simulink library "halout"  (R2021b)
settings: Solver=VariableStepAuto  StartTime=0.0  StopTime=10.0  RelTol=1e-3
undefined symbols (not defined in the file): C_TASK_5MS_S, FALSE, KHAL_CAN1TxReq_flg, KHAL_CAN2TxReq_flg, KHAL_CAN3FD3VCU1toNIDECTxReq_flg, KHAL_CAN3FD3VCU1TxReq_flg, KHAL_CAN3FD3VCU2E2E_flg, KHAL_CAN3FD3VCU2toNIDECE2E_flg, KHAL_CAN3FD3VCU2toNIDECTxReq_flg, KHAL_CAN3FD3VCU2TxReq_flg, KHAL_CAN3TxReq_flg, KHAL_CAN4FD4CE1000E2E_flg, KHAL_CAN4FD4CE1000TxReq_flg, KHAL_CAN4TxReq_flg, KHAL_CAN5TxReq_flg, KHAL_CAN7TxReq_flg, ONE_INT, TRUE, ZERO_INT
libraries: FVT_lib x258, simulink x115
(part 5 of 17)

== system halout/HAL_OUT/CAN3/FD3_THCM1_0x182 ==
  BSCP_outputs : Inport  OutDataTypeStr=Bus: BSCP_outputs
  BOUTP_outputs : Inport  Port=2  OutDataTypeStr=Bus: BOUTP_outputs
  BatteryMode : Subsystem
  CCUACLampSts : Subsystem
  CCUACMaxLampSts : Subsystem
  CCUAutoLampSts : Subsystem
  CCUAutoMidLampSts : Subsystem
  CCUDispalyRequest : Subsystem
  CCUEcoSts : Subsystem
  CCUFrtOnOffLampSts : Subsystem
  CCUHEATMaxLampSts : Subsystem
  CCURrOnOffLampSts : Subsystem
  CCUSyncLampSts : Subsystem
  CabinMode : Subsystem
  EDriveMode : Subsystem
  FDAGSCmd : Subsystem
  FDRecyAutoCmd : Subsystem
  FrCoolantflow : Subsystem
  FrCoolanttemp : Subsystem
  Ground{,1..17} (18 alike) : Ground
  HPThermalRecoveryReq : Subsystem
  RrCoolantflow : Subsystem
  RrCoolanttemp : Subsystem
  bus_creator : BusCreator  Inputs=37  OutDataTypeStr=Bus: DT_CAN3_SG_FD3_THCM1  NonVirtualBus=on
  bus_selector : BusSelector  OutputSignals=VOUTP_BatteryMode_enum
  bus_selector1 : BusSelector  OutputSignals=VOUTP_CCUACLampSts_flg
  bus_selector10 : BusSelector  OutputSignals=VOUTP_sigAmbAirT_C
  bus_selector11 : BusSelector  OutputSignals=VOUTP_sigCbnAirT_C
  bus_selector12 : BusSelector  OutputSignals=VOUTP_sigCbnSolarLeft_W
  bus_selector13 : BusSelector  OutputSignals=VOUTP_sigCbnSolarRight_W
  bus_selector14 : BusSelector  OutputSignals=VOUTP_sigClntTHvBattOut_C
  bus_selector15 : BusSelector  OutputSignals=VOUTP_sigRecircSt_flg
  bus_selector16 : BusSelector  OutputSignals=VOUTP_sigSetTempZon1St_C
  bus_selector17 : BusSelector  OutputSignals=VOUTP_sigSetTempZon2St_C
  bus_selector18 : BusSelector  OutputSignals=VOUTP_sigWindDirZon1St_enum
  bus_selector2 : BusSelector  OutputSignals=VOUTP_CCUACMaxLampSts_flg
  bus_selector3 : BusSelector  OutputSignals=VOUTP_CCUAutoLampSts_flg
  bus_selector4 : BusSelector  OutputSignals=VOUTP_CCUSyncLampSts_flg
  bus_selector5 : BusSelector  OutputSignals=VOUTP_CabinMode_enum
  bus_selector6 : BusSelector  OutputSignals=VOUTP_EDriveMode_enum
  bus_selector7 : BusSelector  OutputSignals=VOUTP_FDAGSCmd_enum
  bus_selector8 : BusSelector  OutputSignals=VOUTP_FDRecyAutoCmd_enum
  bus_selector9 : BusSelector  OutputSignals=VOUTP_sigAirIntenZon1St_enum
  sigAirIntenZon1St : Subsystem
  sigAirIntenZon3St : Subsystem
  sigAmbAirT : Subsystem
  sigCbnAirT : Subsystem
  sigCbnPTCPwrAct : Subsystem
  sigCbnSolarLeft : Subsystem
  sigCbnSolarRight : Subsystem
  sigClmtCmprPwrAct : Subsystem
  sigClntTHvBattOut : Subsystem
  sigDfrstSt : Subsystem
  sigHvacSt : Subsystem
  sigRecircSt : Subsystem
  sigSetTempZon1St : Subsystem
  sigSetTempZon2St : Subsystem
  sigSetTempZon3St : Subsystem
  sigWindDirZon1St : Subsystem
  sigWindDirZon3St : Subsystem
  FD3_THCM1 : Outport
  wires:
  BSCP_outputs/1 -> [BSCP_outputs]
  BOUTP_outputs/1 -> [BOUTP_outputs]
  [CAN3_BatteryMode] -> bus_creator/1  "CAN3_BatteryMode"
  [CAN3_CCU_ACLampSts] -> bus_creator/2  "CAN3_CCU_ACLampSts"
  [CAN3_CCU_ACMaxLampSts] -> bus_creator/3  "CAN3_CCU_ACMaxLampSts"
  [CAN3_CCU_AutoLampSts] -> bus_creator/4  "CAN3_CCU_AutoLampSts"
  [CAN3_CCU_AutoMidLampSts] -> bus_creator/5  "CAN3_CCU_AutoMidLampSts"
  [CAN3_CCU_Dispaly_Request] -> bus_creator/6  "CAN3_CCU_Dispaly_Request"
  [CAN3_CCU_EcoSts] -> bus_creator/7  "CAN3_CCU_EcoSts"
  [CAN3_CCU_FrtOnOffLampSts] -> bus_creator/8  "CAN3_CCU_FrtOnOffLampSts"
  [CAN3_CCU_HEATMaxLampSts] -> bus_creator/9  "CAN3_CCU_HEATMaxLampSts"
  [CAN3_CCU_RrOnOffLampSts] -> bus_creator/10  "CAN3_CCU_RrOnOffLampSts"
  [CAN3_CCU_SyncLampSts] -> bus_creator/11  "CAN3_CCU_SyncLampSts"
  [CAN3_CabinMode] -> bus_creator/12  "CAN3_CabinMode"
  [CAN3_EDriveMode] -> bus_creator/13  "CAN3_EDriveMode"
  [CAN3_FD_AGS_Cmd] -> bus_creator/14  "CAN3_FD_AGS_Cmd"
  [CAN3_FD_RecyAuto_Cmd] -> bus_creator/15  "CAN3_FD_RecyAuto_Cmd"
  [CAN3_Fr_Coolantflow] -> bus_creator/16  "CAN3_Fr_Coolantflow"
  [CAN3_Fr_Coolanttemp] -> bus_creator/17  "CAN3_Fr_Coolanttemp"
  [CAN3_HPThermalRecoveryReq] -> bus_creator/18  "CAN3_HPThermalRecoveryReq"
  [CAN3_Rr_Coolantflow] -> bus_creator/19  "CAN3_Rr_Coolantflow"
  [CAN3_Rr_Coolanttemp] -> bus_creator/20  "CAN3_Rr_Coolanttemp"
  [CAN3_sigAirIntenZon1St] -> bus_creator/21  "CAN3_sigAirIntenZon1St"
  [CAN3_sigAirIntenZon3St] -> bus_creator/22  "CAN3_sigAirIntenZon3St"
  [CAN3_sigAmbAirT] -> bus_creator/23  "CAN3_sigAmbAirT"
  [CAN3_sigCbnAirT] -> bus_creator/24  "CAN3_sigCbnAirT"
  [CAN3_sigCbnPTCPwrAct] -> bus_creator/25  "CAN3_sigCbnPTCPwrAct"
  [CAN3_sigCbnSolarLeft] -> bus_creator/26  "CAN3_sigCbnSolarLeft"
  [CAN3_sigCbnSolarRight] -> bus_creator/27  "CAN3_sigCbnSolarRight"
  [CAN3_sigClmtCmprPwrAct] -> bus_creator/28  "CAN3_sigClmtCmprPwrAct"
  [CAN3_sigClntTHvBattOut] -> bus_creator/29  "CAN3_sigClntTHvBattOut"
  [CAN3_sigDfrstSt] -> bus_creator/30  "CAN3_sigDfrstSt"
  [CAN3_sigHvacSt] -> bus_creator/31  "CAN3_sigHvacSt"
  [CAN3_sigRecircSt] -> bus_creator/32  "CAN3_sigRecircSt"
  [CAN3_sigSetTempZon1St] -> bus_creator/33  "CAN3_sigSetTempZon1St"
  [CAN3_sigSetTempZon2St] -> bus_creator/34  "CAN3_sigSetTempZon2St"
  [CAN3_sigSetTempZon3St] -> bus_creator/35  "CAN3_sigSetTempZon3St"
  [CAN3_sigWindDirZon1St] -> bus_creator/36  "CAN3_sigWindDirZon1St"
  [CAN3_sigWindDirZon3St] -> bus_creator/37  "CAN3_sigWindDirZon3St"
  bus_creator/1 -> FD3_THCM1/1
  BatteryMode/1(CAN3_BatteryMode) -> [CAN3_BatteryMode]
  CCUACLampSts/1(CAN3_CCU_ACLampSts) -> [CAN3_CCU_ACLampSts]
  CCUACMaxLampSts/1(CAN3_CCU_ACMaxLampSts) -> [CAN3_CCU_ACMaxLampSts]
  CCUAutoLampSts/1(CAN3_CCU_AutoLampSts) -> [CAN3_CCU_AutoLampSts]
  CCUAutoMidLampSts/1(CAN3_CCU_AutoMidLampSts) -> [CAN3_CCU_AutoMidLampSts]
  CCUDispalyRequest/1(CAN3_CCU_Dispaly_Request) -> [CAN3_CCU_Dispaly_Request]
  CCUEcoSts/1(CAN3_CCU_EcoSts) -> [CAN3_CCU_EcoSts]
  CCUFrtOnOffLampSts/1(CAN3_CCU_FrtOnOffLampSts) -> [CAN3_CCU_FrtOnOffLampSts]
  CCUHEATMaxLampSts/1(CAN3_CCU_HEATMaxLampSts) -> [CAN3_CCU_HEATMaxLampSts]
  CCURrOnOffLampSts/1(CAN3_CCU_RrOnOffLampSts) -> [CAN3_CCU_RrOnOffLampSts]
  CCUSyncLampSts/1(CAN3_CCU_SyncLampSts) -> [CAN3_CCU_SyncLampSts]
  CabinMode/1(CAN3_CabinMode) -> [CAN3_CabinMode]
  EDriveMode/1(CAN3_EDriveMode) -> [CAN3_EDriveMode]
  FDAGSCmd/1(CAN3_FD_AGS_Cmd) -> [CAN3_FD_AGS_Cmd]
  FDRecyAutoCmd/1(CAN3_FD_RecyAuto_Cmd) -> [CAN3_FD_RecyAuto_Cmd]
  FrCoolantflow/1(CAN3_Fr_Coolantflow) -> [CAN3_Fr_Coolantflow]
  FrCoolanttemp/1(CAN3_Fr_Coolanttemp) -> [CAN3_Fr_Coolanttemp]
  HPThermalRecoveryReq/1(CAN3_HPThermalRecoveryReq) -> [CAN3_HPThermalRecoveryReq]
  RrCoolantflow/1(CAN3_Rr_Coolantflow) -> [CAN3_Rr_Coolantflow]
  RrCoolanttemp/1(CAN3_Rr_Coolanttemp) -> [CAN3_Rr_Coolanttemp]
  sigAirIntenZon1St/1(CAN3_sigAirIntenZon1St) -> [CAN3_sigAirIntenZon1St]
  sigAirIntenZon3St/1(CAN3_sigAirIntenZon3St) -> [CAN3_sigAirIntenZon3St]
  sigAmbAirT/1(CAN3_sigAmbAirT) -> [CAN3_sigAmbAirT]
  sigCbnAirT/1(CAN3_sigCbnAirT) -> [CAN3_sigCbnAirT]
  sigCbnPTCPwrAct/1(CAN3_sigCbnPTCPwrAct) -> [CAN3_sigCbnPTCPwrAct]
  sigCbnSolarLeft/1(CAN3_sigCbnSolarLeft) -> [CAN3_sigCbnSolarLeft]
  sigCbnSolarRight/1(CAN3_sigCbnSolarRight) -> [CAN3_sigCbnSolarRight]
  sigClmtCmprPwrAct/1(CAN3_sigClmtCmprPwrAct) -> [CAN3_sigClmtCmprPwrAct]
  sigClntTHvBattOut/1(CAN3_sigClntTHvBattOut) -> [CAN3_sigClntTHvBattOut]
  sigDfrstSt/1(CAN3_sigDfrstSt) -> [CAN3_sigDfrstSt]
  sigHvacSt/1(CAN3_sigHvacSt) -> [CAN3_sigHvacSt]
  sigRecircSt/1(CAN3_sigRecircSt) -> [CAN3_sigRecircSt]
  sigSetTempZon1St/1(CAN3_sigSetTempZon1St) -> [CAN3_sigSetTempZon1St]
  sigSetTempZon2St/1(CAN3_sigSetTempZon2St) -> [CAN3_sigSetTempZon2St]
  sigSetTempZon3St/1(CAN3_sigSetTempZon3St) -> [CAN3_sigSetTempZon3St]
  sigWindDirZon1St/1(CAN3_sigWindDirZon1St) -> [CAN3_sigWindDirZon1St]
  sigWindDirZon3St/1(CAN3_sigWindDirZon3St) -> [CAN3_sigWindDirZon3St]
  bus_selector/1 -> BatteryMode/1(BatteryMode)  "<VOUTP_BatteryMode_enum>"
  [BOUTP_outputs] -> bus_selector/1
  bus_selector1/1 -> CCUACLampSts/1(CCUACLampSts)  "<VOUTP_CCUACLampSts_flg>"
  [BOUTP_outputs] -> bus_selector1/1
  bus_selector2/1 -> CCUACMaxLampSts/1(CCUACMaxLampSts)  "<VOUTP_CCUACMaxLampSts_flg>"
  [BOUTP_outputs] -> bus_selector2/1
  bus_selector3/1 -> CCUAutoLampSts/1(CCUAutoLampSts)  "<VOUTP_CCUAutoLampSts_flg>"
  [BOUTP_outputs] -> bus_selector3/1
  Ground/1 -> CCUAutoMidLampSts/1(CCUAutoMidLampSts)
  Ground1/1 -> CCUDispalyRequest/1(CCUDispalyRequest)
  Ground2/1 -> CCUEcoSts/1(CCUEcoSts)
  Ground3/1 -> CCUFrtOnOffLampSts/1(CCUFrtOnOffLampSts)
  Ground4/1 -> CCUHEATMaxLampSts/1(CCUHEATMaxLampSts)
  Ground5/1 -> CCURrOnOffLampSts/1(CCURrOnOffLampSts)
  bus_selector4/1 -> CCUSyncLampSts/1(CCUSyncLampSts)  "<VOUTP_CCUSyncLampSts_flg>"
  [BOUTP_outputs] -> bus_selector4/1
  bus_selector5/1 -> CabinMode/1(CabinMode)  "<VOUTP_CabinMode_enum>"
  [BOUTP_outputs] -> bus_selector5/1
  bus_selector6/1 -> EDriveMode/1(EDriveMode)  "<VOUTP_EDriveMode_enum>"
  [BOUTP_outputs] -> bus_selector6/1
  bus_selector7/1 -> FDAGSCmd/1(FDAGSCmd)  "<VOUTP_FDAGSCmd_enum>"
  [BOUTP_outputs] -> bus_selector7/1
  bus_selector8/1 -> FDRecyAutoCmd/1(FDRecyAutoCmd)  "<VOUTP_FDRecyAutoCmd_enum>"
  [BOUTP_outputs] -> bus_selector8/1
  Ground6/1 -> FrCoolantflow/1(FrCoolantflow)
  Ground7/1 -> FrCoolanttemp/1(FrCoolanttemp)
  Ground8/1 -> HPThermalRecoveryReq/1(HPThermalRecoveryReq)
  Ground9/1 -> RrCoolantflow/1(RrCoolantflow)
  Ground10/1 -> RrCoolanttemp/1(RrCoolanttemp)
  bus_selector9/1 -> sigAirIntenZon1St/1(sigAirIntenZon1St)  "<VOUTP_sigAirIntenZon1St_enum>"
  [BOUTP_outputs] -> bus_selector9/1
  Ground11/1 -> sigAirIntenZon3St/1(sigAirIntenZon3St)
  bus_selector10/1 -> sigAmbAirT/1(sigAmbAirT)  "<VOUTP_sigAmbAirT_C>"
  [BOUTP_outputs] -> bus_selector10/1
  bus_selector11/1 -> sigCbnAirT/1(sigCbnAirT)  "<VOUTP_sigCbnAirT_C>"
  [BOUTP_outputs] -> bus_selector11/1
  Ground12/1 -> sigCbnPTCPwrAct/1(sigCbnPTCPwrAct)
  bus_selector12/1 -> sigCbnSolarLeft/1(sigCbnSolarLeft)  "<VOUTP_sigCbnSolarLeft_W>"
  [BOUTP_outputs] -> bus_selector12/1
  bus_selector13/1 -> sigCbnSolarRight/1(sigCbnSolarRight)  "<VOUTP_sigCbnSolarRight_W>"
  [BOUTP_outputs] -> bus_selector13/1
  Ground13/1 -> sigClmtCmprPwrAct/1(sigClmtCmprPwrAct)
  bus_selector14/1 -> sigClntTHvBattOut/1(sigClntTHvBattOut)  "<VOUTP_sigClntTHvBattOut_C>"
  [BOUTP_outputs] -> bus_selector14/1
  Ground14/1 -> sigDfrstSt/1(sigDfrstSt)
  Ground15/1 -> sigHvacSt/1(sigHvacSt)
  bus_selector15/1 -> sigRecircSt/1(sigRecircSt)  "<VOUTP_sigRecircSt_flg>"
  [BOUTP_outputs] -> bus_selector15/1
  bus_selector16/1 -> sigSetTempZon1St/1(sigSetTempZon1St)  "<VOUTP_sigSetTempZon1St_C>"
  [BOUTP_outputs] -> bus_selector16/1
  bus_selector17/1 -> sigSetTempZon2St/1(sigSetTempZon2St)  "<VOUTP_sigSetTempZon2St_C>"
  [BOUTP_outputs] -> bus_selector17/1
  Ground16/1 -> sigSetTempZon3St/1(sigSetTempZon3St)
  bus_selector18/1 -> sigWindDirZon1St/1(sigWindDirZon1St)  "<VOUTP_sigWindDirZon1St_enum>"
  [BOUTP_outputs] -> bus_selector18/1
  Ground17/1 -> sigWindDirZon3St/1(sigWindDirZon3St)

== system halout/HAL_OUT/CAN3/FD3_THCM2_0x186 ==
  BSCP_outputs : Inport  OutDataTypeStr=Bus: BSCP_outputs
  BOUTP_outputs : Inport  Port=2  OutDataTypeStr=Bus: BOUTP_outputs
  ACSubMode : Subsystem
  APTCActFrRiPwr : Subsystem
  BatLoopActWtFlw : Subsystem
  CCUCbnPreACWkSts : Subsystem
  CCUCbnPreEstimdTi : Subsystem
  CCUCbnPreSts : Subsystem
  CCUHiVoltageReq : Subsystem
  CoolgFanActDuty : Subsystem
  DeiceModReq : Subsystem
  FDBlowerCmd : Subsystem
  FDCompCmd : Subsystem
  FDEWP1Cmd : Subsystem
  FDEWP2Cmd : Subsystem
  FDEWP3Cmd : Subsystem
  FDEXV1Cmd : Subsystem
  FDEXV2Cmd : Subsystem
  FDFWVCmd : Subsystem
  FDFrLeAPTCHeatPwrCmd : Subsystem
  FDFrRiAPTCHeatPwrCmd : Subsystem
  FDFrWPTCHeatPwrCmd : Subsystem
  FDRrAPTCHeatPwrCmd : Subsystem
  FDSOTXVCmd : Subsystem
  FDSOV1Cmd : Subsystem
  FDSOV2Cmd : Subsystem
  FDSOV3Cmd : Subsystem
  FDTWVCmd : Subsystem
  Ground{,1..6} (7 alike) : Ground
  bus_creator : BusCreator  Inputs=26  OutDataTypeStr=Bus: DT_CAN3_SG_FD3_THCM2  NonVirtualBus=on
  bus_selector : BusSelector  OutputSignals=VOUTP_ACSubMode_enum
  bus_selector1 : BusSelector  OutputSignals=VOUTP_CoolgFanActDuty_pct
  bus_selector10 : BusSelector  OutputSignals=VOUTP_FDFrLeAPTCHeatPwrCmd_W
  bus_selector11 : BusSelector  OutputSignals=VOUTP_FDFrRiAPTCHeatPwrCmd_W
  bus_selector12 : BusSelector  OutputSignals=VOUTP_FDFrWPTCHeatPwrCmd_W
  bus_selector13 : BusSelector  OutputSignals=VOUTP_FDRrAPTCHeatPwrCmd_W
  bus_selector14 : BusSelector  OutputSignals=VOUTP_FDSOTXVCmd_flg
  bus_selector15 : BusSelector  OutputSignals=VOUTP_FDSOV1Cmd_flg
  bus_selector16 : BusSelector  OutputSignals=VOUTP_FDSOV2Cmd_flg
  bus_selector17 : BusSelector  OutputSignals=VOUTP_FDSOV3Cmd_flg
  bus_selector18 : BusSelector  OutputSignals=VOUTP_FDTWVCmd_pct
  bus_selector2 : BusSelector  OutputSignals=VOUTP_FDBlowerCmd_pct
  bus_selector3 : BusSelector  OutputSignals=VOUTP_FDCompCmd_rpm
  bus_selector4 : BusSelector  OutputSignals=VOUTP_FDEWP1Cmd_enum
  bus_selector5 : BusSelector  OutputSignals=VOUTP_FDEWP2Cmd_enum
  bus_selector6 : BusSelector  OutputSignals=VOUTP_FDEWP3Cmd_enum
  bus_selector7 : BusSelector  OutputSignals=VOUTP_FDEXV1Cmd_step
  bus_selector8 : BusSelector  OutputSignals=VOUTP_FDEXV2Cmd_step
  bus_selector9 : BusSelector  OutputSignals=VOUTP_FDFWVCmd_flg
  FD3_THCM2 : Outport
  wires:
  BSCP_outputs/1 -> [BSCP_outputs]
  BOUTP_outputs/1 -> [BOUTP_outputs]
  [CAN3_ACSubMode] -> bus_creator/1  "CAN3_ACSubMode"
  [CAN3_APTC_ActFrRiPwr] -> bus_creator/2  "CAN3_APTC_ActFrRiPwr"
  [CAN3_BatLoopActWtFlw] -> bus_creator/3  "CAN3_BatLoopActWtFlw"
  [CAN3_CCU_CbnPreACWkSts] -> bus_creator/4  "CAN3_CCU_CbnPreACWkSts"
  [CAN3_CCU_CbnPreEstimdTi] -> bus_creator/5  "CAN3_CCU_CbnPreEstimdTi"
  [CAN3_CCU_CbnPreSts] -> bus_creator/6  "CAN3_CCU_CbnPreSts"
  [CAN3_CCU_HiVoltageReq] -> bus_creator/7  "CAN3_CCU_HiVoltageReq"
  [CAN3_CoolgFanActDuty] -> bus_creator/8  "CAN3_CoolgFanActDuty"
  [CAN3_DeiceModReq] -> bus_creator/9  "CAN3_DeiceModReq"
  [CAN3_FD_Blower_Cmd] -> bus_creator/10  "CAN3_FD_Blower_Cmd"
  [CAN3_FD_Comp_Cmd] -> bus_creator/11  "CAN3_FD_Comp_Cmd"
  [CAN3_FD_EWP1_Cmd] -> bus_creator/12  "CAN3_FD_EWP1_Cmd"
  [CAN3_FD_EWP2_Cmd] -> bus_creator/13  "CAN3_FD_EWP2_Cmd"
  [CAN3_FD_EWP3_Cmd] -> bus_creator/14  "CAN3_FD_EWP3_Cmd"
  [CAN3_FD_EXV1_Cmd] -> bus_creator/15  "CAN3_FD_EXV1_Cmd"
  [CAN3_FD_EXV2_Cmd] -> bus_creator/16  "CAN3_FD_EXV2_Cmd"
  [CAN3_FD_FWV_Cmd] -> bus_creator/17  "CAN3_FD_FWV_Cmd"
  [CAN3_FD_FrLeAPTCHeatPwr_Cmd] -> bus_creator/18  "CAN3_FD_FrLeAPTCHeatPwr_Cmd"
  [CAN3_FD_FrRiAPTCHeatPwr_Cmd] -> bus_creator/19  "CAN3_FD_FrRiAPTCHeatPwr_Cmd"
  [CAN3_FD_FrWPTCHeatPwr_Cmd] -> bus_creator/20  "CAN3_FD_FrWPTCHeatPwr_Cmd"
  [CAN3_FD_RrAPTCHeatPwr_Cmd] -> bus_creator/21  "CAN3_FD_RrAPTCHeatPwr_Cmd"
  [CAN3_FD_SOTXV_Cmd] -> bus_creator/22  "CAN3_FD_SOTXV_Cmd"
  [CAN3_FD_SOV1_Cmd] -> bus_creator/23  "CAN3_FD_SOV1_Cmd"
  [CAN3_FD_SOV2_Cmd] -> bus_creator/24  "CAN3_FD_SOV2_Cmd"
  [CAN3_FD_SOV3_Cmd] -> bus_creator/25  "CAN3_FD_SOV3_Cmd"
  [CAN3_FD_TWV_Cmd] -> bus_creator/26  "CAN3_FD_TWV_Cmd"
  bus_creator/1 -> FD3_THCM2/1
  ACSubMode/1(CAN3_ACSubMode) -> [CAN3_ACSubMode]
  APTCActFrRiPwr/1(CAN3_APTC_ActFrRiPwr) -> [CAN3_APTC_ActFrRiPwr]
  BatLoopActWtFlw/1(CAN3_BatLoopActWtFlw) -> [CAN3_BatLoopActWtFlw]
  CCUCbnPreACWkSts/1(CAN3_CCU_CbnPreACWkSts) -> [CAN3_CCU_CbnPreACWkSts]
  CCUCbnPreEstimdTi/1(CAN3_CCU_CbnPreEstimdTi) -> [CAN3_CCU_CbnPreEstimdTi]
  CCUCbnPreSts/1(CAN3_CCU_CbnPreSts) -> [CAN3_CCU_CbnPreSts]
  CCUHiVoltageReq/1(CAN3_CCU_HiVoltageReq) -> [CAN3_CCU_HiVoltageReq]
  CoolgFanActDuty/1(CAN3_CoolgFanActDuty) -> [CAN3_CoolgFanActDuty]
  DeiceModReq/1(CAN3_DeiceModReq) -> [CAN3_DeiceModReq]
  FDBlowerCmd/1(CAN3_FD_Blower_Cmd) -> [CAN3_FD_Blower_Cmd]
  FDCompCmd/1(CAN3_FD_Comp_Cmd) -> [CAN3_FD_Comp_Cmd]
  FDEWP1Cmd/1(CAN3_FD_EWP1_Cmd) -> [CAN3_FD_EWP1_Cmd]
  FDEWP2Cmd/1(CAN3_FD_EWP2_Cmd) -> [CAN3_FD_EWP2_Cmd]
  FDEWP3Cmd/1(CAN3_FD_EWP3_Cmd) -> [CAN3_FD_EWP3_Cmd]
  FDEXV1Cmd/1(CAN3_FD_EXV1_Cmd) -> [CAN3_FD_EXV1_Cmd]
  FDEXV2Cmd/1(CAN3_FD_EXV2_Cmd) -> [CAN3_FD_EXV2_Cmd]
  FDFWVCmd/1(CAN3_FD_FWV_Cmd) -> [CAN3_FD_FWV_Cmd]
  FDFrLeAPTCHeatPwrCmd/1(CAN3_FD_FrLeAPTCHeatPwr_Cmd) -> [CAN3_FD_FrLeAPTCHeatPwr_Cmd]
  FDFrRiAPTCHeatPwrCmd/1(CAN3_FD_FrRiAPTCHeatPwr_Cmd) -> [CAN3_FD_FrRiAPTCHeatPwr_Cmd]
  FDFrWPTCHeatPwrCmd/1(CAN3_FD_FrWPTCHeatPwr_Cmd) -> [CAN3_FD_FrWPTCHeatPwr_Cmd]
  FDRrAPTCHeatPwrCmd/1(CAN3_FD_RrAPTCHeatPwr_Cmd) -> [CAN3_FD_RrAPTCHeatPwr_Cmd]
  FDSOTXVCmd/1(CAN3_FD_SOTXV_Cmd) -> [CAN3_FD_SOTXV_Cmd]
  FDSOV1Cmd/1(CAN3_FD_SOV1_Cmd) -> [CAN3_FD_SOV1_Cmd]
  FDSOV2Cmd/1(CAN3_FD_SOV2_Cmd) -> [CAN3_FD_SOV2_Cmd]
  FDSOV3Cmd/1(CAN3_FD_SOV3_Cmd) -> [CAN3_FD_SOV3_Cmd]
  FDTWVCmd/1(CAN3_FD_TWV_Cmd) -> [CAN3_FD_TWV_Cmd]
  bus_selector/1 -> ACSubMode/1(ACSubMode)  "<VOUTP_ACSubMode_enum>"
  [BOUTP_outputs] -> bus_selector/1
  Ground/1 -> APTCActFrRiPwr/1(APTCActFrRiPwr)
  Ground1/1 -> BatLoopActWtFlw/1(BatLoopActWtFlw)
  Ground2/1 -> CCUCbnPreACWkSts/1(CCUCbnPreACWkSts)
  Ground3/1 -> CCUCbnPreEstimdTi/1(CCUCbnPreEstimdTi)
  Ground4/1 -> CCUCbnPreSts/1(CCUCbnPreSts)
  Ground5/1 -> CCUHiVoltageReq/1(CCUHiVoltageReq)
  bus_selector1/1 -> CoolgFanActDuty/1(CoolgFanActDuty)  "<VOUTP_CoolgFanActDuty_pct>"
  [BOUTP_outputs] -> bus_selector1/1
  Ground6/1 -> DeiceModReq/1(DeiceModReq)
  bus_selector2/1 -> FDBlowerCmd/1(FDBlowerCmd)  "<VOUTP_FDBlowerCmd_pct>"
  [BOUTP_outputs] -> bus_selector2/1
  bus_selector3/1 -> FDCompCmd/1(FDCompCmd)  "<VOUTP_FDCompCmd_rpm>"
  [BOUTP_outputs] -> bus_selector3/1
  bus_selector4/1 -> FDEWP1Cmd/1(FDEWP1Cmd)  "<VOUTP_FDEWP1Cmd_enum>"
  [BOUTP_outputs] -> bus_selector4/1
  bus_selector5/1 -> FDEWP2Cmd/1(FDEWP2Cmd)  "<VOUTP_FDEWP2Cmd_enum>"
  [BOUTP_outputs] -> bus_selector5/1
  bus_selector6/1 -> FDEWP3Cmd/1(FDEWP3Cmd)  "<VOUTP_FDEWP3Cmd_enum>"
  [BOUTP_outputs] -> bus_selector6/1
  bus_selector7/1 -> FDEXV1Cmd/1(FDEXV1Cmd)  "<VOUTP_FDEXV1Cmd_step>"
  [BOUTP_outputs] -> bus_selector7/1
  bus_selector8/1 -> FDEXV2Cmd/1(FDEXV2Cmd)  "<VOUTP_FDEXV2Cmd_step>"
  [BOUTP_outputs] -> bus_selector8/1
  bus_selector9/1 -> FDFWVCmd/1(FDFWVCmd)  "<VOUTP_FDFWVCmd_flg>"
  [BOUTP_outputs] -> bus_selector9/1
  bus_selector10/1 -> FDFrLeAPTCHeatPwrCmd/1(FDFrLeAPTCHeatPwrCmd)  "<VOUTP_FDFrLeAPTCHeatPwrCmd_W>"
  [BOUTP_outputs] -> bus_selector10/1
  bus_selector11/1 -> FDFrRiAPTCHeatPwrCmd/1(FDFrRiAPTCHeatPwrCmd)  "<VOUTP_FDFrRiAPTCHeatPwrCmd_W>"
  [BOUTP_outputs] -> bus_selector11/1
  bus_selector12/1 -> FDFrWPTCHeatPwrCmd/1(FDFrWPTCHeatPwrCmd)  "<VOUTP_FDFrWPTCHeatPwrCmd_W>"
  [BOUTP_outputs] -> bus_selector12/1
  bus_selector13/1 -> FDRrAPTCHeatPwrCmd/1(FDRrAPTCHeatPwrCmd)  "<VOUTP_FDRrAPTCHeatPwrCmd_W>"
  [BOUTP_outputs] -> bus_selector13/1
  bus_selector14/1 -> FDSOTXVCmd/1(FDSOTXVCmd)  "<VOUTP_FDSOTXVCmd_flg>"
  [BOUTP_outputs] -> bus_selector14/1
  bus_selector15/1 -> FDSOV1Cmd/1(FDSOV1Cmd)  "<VOUTP_FDSOV1Cmd_flg>"
  [BOUTP_outputs] -> bus_selector15/1
  bus_selector16/1 -> FDSOV2Cmd/1(FDSOV2Cmd)  "<VOUTP_FDSOV2Cmd_flg>"
  [BOUTP_outputs] -> bus_selector16/1
  bus_selector17/1 -> FDSOV3Cmd/1(FDSOV3Cmd)  "<VOUTP_FDSOV3Cmd_flg>"
  [BOUTP_outputs] -> bus_selector17/1
  bus_selector18/1 -> FDTWVCmd/1(FDTWVCmd)  "<VOUTP_FDTWVCmd_pct>"
  [BOUTP_outputs] -> bus_selector18/1

== system halout/HAL_OUT/CAN3/FD3_V2L1_0x374 ==
  BSCP_outputs : Inport  OutDataTypeStr=Bus: BSCP_outputs
  BOUTP_outputs : Inport  Port=2  OutDataTypeStr=Bus: BOUTP_outputs
  Ground : Ground
  ReqOBCV2LEna : Subsystem
  ReqV2LIVIPopup : Subsystem
  ReqV2LSwOn : Subsystem
  bus_creator : BusCreator  Inputs=3  OutDataTypeStr=Bus: DT_CAN3_SG_FD3_V2L1  NonVirtualBus=on
  bus_selector : BusSelector  OutputSignals=VOUTP_ReqOBCV2LEna_enum
  bus_selector1 : BusSelector  OutputSignals=VOUTP_ReqV2LIVIPopup_enum
  FD3_V2L1 : Outport
  wires:
  BSCP_outputs/1 -> [BSCP_outputs]
  BOUTP_outputs/1 -> [BOUTP_outputs]
  [CAN3_Req_OBCV2LEna] -> bus_creator/1  "CAN3_Req_OBCV2LEna"
  [CAN3_Req_V2LSwOn] -> bus_creator/2  "CAN3_Req_V2LSwOn"
  [CAN3_Req_V2L_IVI_Popup] -> bus_creator/3  "CAN3_Req_V2L_IVI_Popup"
  bus_creator/1 -> FD3_V2L1/1
  ReqOBCV2LEna/1(CAN3_Req_OBCV2LEna) -> [CAN3_Req_OBCV2LEna]
  ReqV2LSwOn/1(CAN3_Req_V2LSwOn) -> [CAN3_Req_V2LSwOn]
  ReqV2LIVIPopup/1(CAN3_Req_V2L_IVI_Popup) -> [CAN3_Req_V2L_IVI_Popup]
  bus_selector/1 -> ReqOBCV2LEna/1(ReqOBCV2LEna)  "<VOUTP_ReqOBCV2LEna_enum>"
  [BOUTP_outputs] -> bus_selector/1
  Ground/1 -> ReqV2LSwOn/1(ReqV2LSwOn)
  bus_selector1/1 -> ReqV2LIVIPopup/1(ReqV2LIVIPopup)  "<VOUTP_ReqV2LIVIPopup_enum>"
  [BOUTP_outputs] -> bus_selector1/1

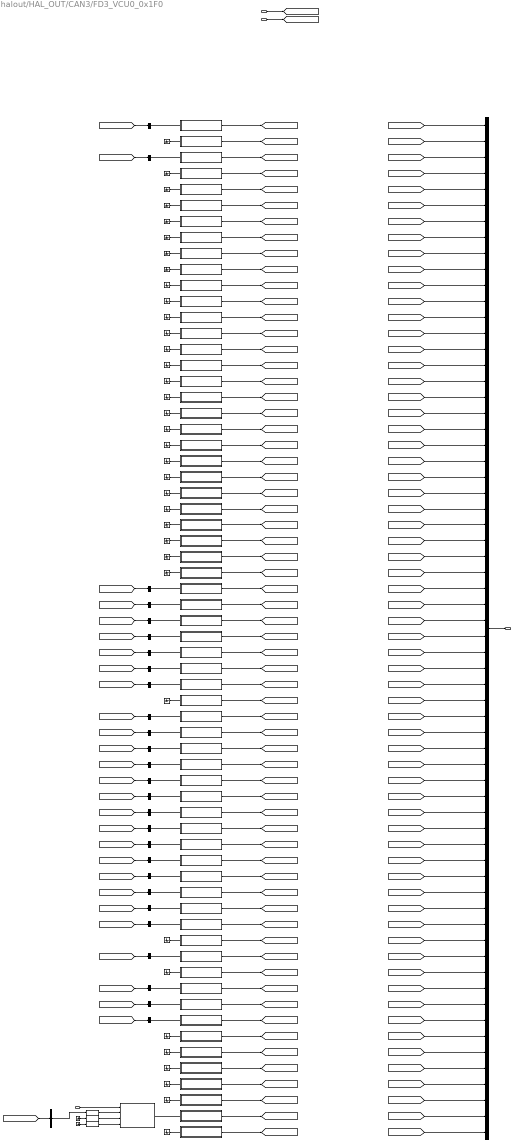
== system halout/HAL_OUT/CAN3/FD3_VCU0_0x1F0 ==
  BSCP_outputs : Inport  OutDataTypeStr=Bus: BSCP_outputs
  BOUTP_outputs : Inport  Port=2  OutDataTypeStr=Bus: BOUTP_outputs
  s8_AcoreReadyToSleep : Inport  Port=3
  Data Type Conversion : DataTypeConversion  OutDataTypeStr=uint8
  Data Type Conversion1 : DataTypeConversion  OutDataTypeStr=uint8
  Data Type Conversion2 : DataTypeConversion  OutDataTypeStr=uint8
  EVCCAplusPwrUpReq : Subsystem
  FDADC12VDet : Subsystem
  FDADC12VDetAvg : Subsystem
  FDCVCUActMaxSlideRateSta : Subsystem
  FDCVCUAllowMovThdOTASta : Subsystem
  FDCVCUDTCCarouselSta : Subsystem
  FDCVCUForcePCmd : Subsystem
  FDCVCUOTAPwrReqOFFChkSta : Subsystem
  FDCVCUOTAPwrReqStdChkSta : Subsystem
  FDCVCUPwrReqOTASta : Subsystem
  FDCVCURWDRDCActiveSta : Subsystem
  FDCVCURegenTqLimitEnSta : Subsystem
  FDCVCUSlideRegenLimTqSta : Subsystem
  FDCVCUVehActSpdSta : Subsystem
  FDCVCUVehMalfunLevelSta : Subsystem
  FDCVMCActStESCYawSta : Subsystem
  FDCVMCLongAccSta : Subsystem
  FUSIONCMM1 : Subsystem
  FUSIONCMM10 : Subsystem
  FUSIONCMM2 : Subsystem
  FUSIONCMM3 : Subsystem
  FUSIONCMM4 : Subsystem
  FUSIONCMM5 : Subsystem
  FUSIONCMM6 : Subsystem
  FUSIONCMM7 : Subsystem
  FUSIONCMM8 : Subsystem
  FUSIONCMM9 : Subsystem
  FrTqSource : Subsystem
  Ground{,1..37} (38 alike) : Ground
  HVRlyOpFail : Subsystem
  HVTHCMSysAvail : Subsystem
  LVBattChrgtimeAct : Subsystem
  LVBattVoltSta : Subsystem
  LVChrgHoldTAct : Subsystem
  LVSilentChrgLv : Subsystem
  LVSilentChrgReq : Subsystem
  LVSilentChrgSta : Subsystem
  MCUActDisFail : Subsystem
  PMMAllowECUSleep : Subsystem
  PmicBootReason : Subsystem
  PowerDownFault : Subsystem
  PowerDownState : Subsystem
  PowerUpFault : Subsystem
  PowerUpState : Subsystem
  PwrDownReq : Subsystem
  PwrStaConstraint : Subsystem
  PwrStaONTOIVIPopReq : Subsystem
  PwrStaONTOIVIPopT : Subsystem
  PwrStaSelect : Subsystem
  PwrStaTOSta : Subsystem
  PwrUpReq : Subsystem
  RrTqSource : Subsystem
  SchedChgTOSta : Subsystem
  SilentChkAllowSleep : Subsystem
  Subsystem : Subsystem
  SysAllowReadySta : Subsystem
  SysPwrSta : Subsystem
  TCountSta : Subsystem
  TimerAllowSleep : Subsystem
  VCUBrkSWSta : Subsystem
  VCUFLDoorSta : Subsystem
  VCUFRDoorSta : Subsystem
  VCURLDoorSta : Subsystem
  VCURRDoorSta : Subsystem
  VehHVPwrAvail4THCM : Subsystem
  WisrBootReason : Subsystem
  bus_creator : BusCreator  Inputs=64  OutDataTypeStr=Bus: DT_CAN3_SG_FD3_VCU0  NonVirtualBus=on
  bus_selector : BusSelector  OutputSignals=VOUTP_EvccAplusPwrUpReq_flg
  bus_selector1 : BusSelector  OutputSignals=VOUTP_FDADC12VDetAvg_mV
  bus_selector10 : BusSelector  OutputSignals=VOUTP_PmicBootReason_enum
  bus_selector11 : BusSelector  OutputSignals=VOUTP_PowerDownFault_enum
  bus_selector12 : BusSelector  OutputSignals=VOUTP_PowerDownState_enum
  bus_selector13 : BusSelector  OutputSignals=VOUTP_PowerUpFault_enum
  bus_selector14 : BusSelector  OutputSignals=VOUTP_PowerUpState_enum
  bus_selector15 : BusSelector  OutputSignals=VOUTP_PwrDownReq_enum
  bus_selector16 : BusSelector  OutputSignals=VOUTP_PwrStaConstraint_enum
  bus_selector17 : BusSelector  OutputSignals=VOUTP_PwrStaONTOPopReq_flg
  bus_selector18 : BusSelector  OutputSignals=VOUTP_IVIPwrStaONTOPopT_s
  bus_selector19 : BusSelector  OutputSignals=VOUTP_PwrStaSelect_enum
  bus_selector2 : BusSelector  OutputSignals=VOUTP_HVTHCMSysAvail_enum
  bus_selector20 : BusSelector  OutputSignals=VOUTP_PwrStaTOSta_enum
  bus_selector21 : BusSelector  OutputSignals=VOUTP_PwrUpReq_enum
  bus_selector22 : BusSelector  OutputSignals=VOUTP_TqSourceRr_enum
  bus_selector23 : BusSelector  OutputSignals=VOUTP_SilentChkAllowSleep_flg
  bus_selector24 : BusSelector  OutputSignals=VOUTP_SysPowerMode_enum
  bus_selector25 : BusSelector  OutputSignals=VOUTP_TCountSta_enum
  bus_selector26 : BusSelector  OutputSignals=VOUTP_TimerAllowSleep_flg
  bus_selector28 : BusSelector  OutputSignals=VOUTP_CurrentNmState_enum
  bus_selector3 : BusSelector  OutputSignals=VOUTP_LVBattChrgTimeCnt_s
  bus_selector4 : BusSelector  OutputSignals=VOUTP_LVBattVoltSta_enum
  bus_selector5 : BusSelector  OutputSignals=VOUTP_LVChrgHoldTtimer_s
  bus_selector6 : BusSelector  OutputSignals=VOUTP_LVSilentChrgLv_enum
  bus_selector7 : BusSelector  OutputSignals=VOUTP_LVSilentChrgReq_flg
  bus_selector8 : BusSelector  OutputSignals=VOUTP_LVSilentChrgSta_enum
  bus_selector9 : BusSelector  OutputSignals=VOUTP_PMMAllowECUSleep_flg
  FD3_VCU0 : Outport
  wires:
  BSCP_outputs/1 -> [BSCP_outputs]
  BOUTP_outputs/1 -> [BOUTP_outputs]
  [CAN3_EVCCAplusPwrUpReq] -> bus_creator/1  "CAN3_EVCCAplusPwrUpReq"
  [CAN3_FDADC12VDet] -> bus_creator/2  "CAN3_FDADC12VDet"
  [CAN3_FDADC12VDetAvg] -> bus_creator/3  "CAN3_FDADC12VDetAvg"
  [CAN3_FDC_VCU_ActMaxSlideRate_Sta] -> bus_creator/4  "CAN3_FDC_VCU_ActMaxSlideRate_Sta"
  [CAN3_FDC_VCU_AllowMovThd_OTA_Sta] -> bus_creator/5  "CAN3_FDC_VCU_AllowMovThd_OTA_Sta"
  [CAN3_FDC_VCU_DTCCarousel_Sta] -> bus_creator/6  "CAN3_FDC_VCU_DTCCarousel_Sta"
  [CAN3_FDC_VCU_ForceP_Cmd] -> bus_creator/7  "CAN3_FDC_VCU_ForceP_Cmd"
  [CAN3_FDC_VCU_OTAPwrReqOFFChk_Sta] -> bus_creator/8  "CAN3_FDC_VCU_OTAPwrReqOFFChk_Sta"
  [CAN3_FDC_VCU_OTAPwrReqStdChk_Sta] -> bus_creator/9  "CAN3_FDC_VCU_OTAPwrReqStdChk_Sta"
  [CAN3_FDC_VCU_PwrReq_OTA_Sta] -> bus_creator/10  "CAN3_FDC_VCU_PwrReq_OTA_Sta"
  [CAN3_FDC_VCU_RWDRDCActive_Sta] -> bus_creator/11  "CAN3_FDC_VCU_RWDRDCActive_Sta"
  [CAN3_FDC_VCU_RegenTqLimitEn_Sta] -> bus_creator/12  "CAN3_FDC_VCU_RegenTqLimitEn_Sta"
  [CAN3_FDC_VCU_SlideRegenLimTq_Sta] -> bus_creator/13  "CAN3_FDC_VCU_SlideRegenLimTq_Sta"
  [CAN3_FDC_VCU_VehActSpd_Sta] -> bus_creator/14  "CAN3_FDC_VCU_VehActSpd_Sta"
  [CAN3_FDC_VCU_VehMalfunLevel_Sta] -> bus_creator/15  "CAN3_FDC_VCU_VehMalfunLevel_Sta"
  [CAN3_FDC_VMC_ActStESCYaw_Sta] -> bus_creator/16  "CAN3_FDC_VMC_ActStESCYaw_Sta"
  [CAN3_FDC_VMC_LongAcc_Sta] -> bus_creator/17  "CAN3_FDC_VMC_LongAcc_Sta"
  [CAN3_FUSION_CMM1] -> bus_creator/18  "CAN3_FUSION_CMM1"
  [CAN3_FUSION_CMM10] -> bus_creator/19  "CAN3_FUSION_CMM10"
  [CAN3_FUSION_CMM2] -> bus_creator/20  "CAN3_FUSION_CMM2"
  [CAN3_FUSION_CMM3] -> bus_creator/21  "CAN3_FUSION_CMM3"
  [CAN3_FUSION_CMM4] -> bus_creator/22  "CAN3_FUSION_CMM4"
  [CAN3_FUSION_CMM5] -> bus_creator/23  "CAN3_FUSION_CMM5"
  [CAN3_FUSION_CMM6] -> bus_creator/24  "CAN3_FUSION_CMM6"
  [CAN3_FUSION_CMM7] -> bus_creator/25  "CAN3_FUSION_CMM7"
  [CAN3_FUSION_CMM8] -> bus_creator/26  "CAN3_FUSION_CMM8"
  [CAN3_FUSION_CMM9] -> bus_creator/27  "CAN3_FUSION_CMM9"
  [CAN3_Fr_TqSource] -> bus_creator/28  "CAN3_Fr_TqSource"
  [CAN3_HVRlyOpFail] -> bus_creator/29  "CAN3_HVRlyOpFail"
  [CAN3_HVTHCMSysAvail] -> bus_creator/30  "CAN3_HVTHCMSysAvail"
  [CAN3_LVBattChrgtimeAct] -> bus_creator/31  "CAN3_LVBattChrgtimeAct"
  [CAN3_LVBattVoltSta] -> bus_creator/32  "CAN3_LVBattVoltSta"
  [CAN3_LVChrgHoldTAct] -> bus_creator/33  "CAN3_LVChrgHoldTAct"
  [CAN3_LVSilentChrgLv] -> bus_creator/34  "CAN3_LVSilentChrgLv"
  [CAN3_LVSilentChrgReq] -> bus_creator/35  "CAN3_LVSilentChrgReq"
  [CAN3_LVSilentChrgSta] -> bus_creator/36  "CAN3_LVSilentChrgSta"
  [CAN3_MCUActDisFail] -> bus_creator/37  "CAN3_MCUActDisFail"
  [CAN3_PMMAllowECUSleep] -> bus_creator/38  "CAN3_PMMAllowECUSleep"
  [CAN3_PmicBootReason] -> bus_creator/39  "CAN3_PmicBootReason"
  [CAN3_PowerDownFault] -> bus_creator/40  "CAN3_PowerDownFault"
  [CAN3_PowerDownState] -> bus_creator/41  "CAN3_PowerDownState"
  [CAN3_PowerUpFault] -> bus_creator/42  "CAN3_PowerUpFault"
  [CAN3_PowerUpState] -> bus_creator/43  "CAN3_PowerUpState"
  [CAN3_PwrDownReq] -> bus_creator/44  "CAN3_PwrDownReq"
  [CAN3_PwrStaConstraint] -> bus_creator/45  "CAN3_PwrStaConstraint"
  [CAN3_PwrStaONTOIVIPopReq] -> bus_creator/46  "CAN3_PwrStaONTOIVIPopReq"
  [CAN3_PwrStaONTOIVIPopT] -> bus_creator/47  "CAN3_PwrStaONTOIVIPopT"
  [CAN3_PwrStaSelect] -> bus_creator/48  "CAN3_PwrStaSelect"
  [CAN3_PwrStaTOSta] -> bus_creator/49  "CAN3_PwrStaTOSta"
  [CAN3_PwrUpReq] -> bus_creator/50  "CAN3_PwrUpReq"
  [CAN3_Rr_TqSource] -> bus_creator/51  "CAN3_Rr_TqSource"
  [CAN3_SchedChgTOSta] -> bus_creator/52  "CAN3_SchedChgTOSta"
  [CAN3_SilentChkAllowSleep] -> bus_creator/53  "CAN3_SilentChkAllowSleep"
  [CAN3_SysAllowReadySta] -> bus_creator/54  "CAN3_SysAllowReadySta"
  [CAN3_SysPwrSta] -> bus_creator/55  "CAN3_SysPwrSta"
  [CAN3_TCountSta] -> bus_creator/56  "CAN3_TCountSta"
  [CAN3_TimerAllowSleep] -> bus_creator/57  "CAN3_TimerAllowSleep"
  [CAN3_VCUBrkSWSta] -> bus_creator/58  "CAN3_VCUBrkSWSta"
  [CAN3_VCUFLDoorSta] -> bus_creator/59  "CAN3_VCUFLDoorSta"
  [CAN3_VCUFRDoorSta] -> bus_creator/60  "CAN3_VCUFRDoorSta"
  [CAN3_VCURLDoorSta] -> bus_creator/61  "CAN3_VCURLDoorSta"
  [CAN3_VCURRDoorSta] -> bus_creator/62  "CAN3_VCURRDoorSta"
  [CAN3_VehHVPwrAvail4THCM] -> bus_creator/63  "CAN3_VehHVPwrAvail4THCM"
  [CAN3_WisrBootReason] -> bus_creator/64  "CAN3_WisrBootReason"
  bus_creator/1 -> FD3_VCU0/1
  EVCCAplusPwrUpReq/1(CAN3_EVCCAplusPwrUpReq) -> [CAN3_EVCCAplusPwrUpReq]
  FDADC12VDet/1(CAN3_FDADC12VDet) -> [CAN3_FDADC12VDet]
  FDADC12VDetAvg/1(CAN3_FDADC12VDetAvg) -> [CAN3_FDADC12VDetAvg]
  FDCVCUActMaxSlideRateSta/1(CAN3_FDC_VCU_ActMaxSlideRate_Sta) -> [CAN3_FDC_VCU_ActMaxSlideRate_Sta]
  FDCVCUAllowMovThdOTASta/1(CAN3_FDC_VCU_AllowMovThd_OTA_Sta) -> [CAN3_FDC_VCU_AllowMovThd_OTA_Sta]
  FDCVCUDTCCarouselSta/1(CAN3_FDC_VCU_DTCCarousel_Sta) -> [CAN3_FDC_VCU_DTCCarousel_Sta]
  FDCVCUForcePCmd/1(CAN3_FDC_VCU_ForceP_Cmd) -> [CAN3_FDC_VCU_ForceP_Cmd]
  FDCVCUOTAPwrReqOFFChkSta/1(CAN3_FDC_VCU_OTAPwrReqOFFChk_Sta) -> [CAN3_FDC_VCU_OTAPwrReqOFFChk_Sta]
  FDCVCUOTAPwrReqStdChkSta/1(CAN3_FDC_VCU_OTAPwrReqStdChk_Sta) -> [CAN3_FDC_VCU_OTAPwrReqStdChk_Sta]
  FDCVCUPwrReqOTASta/1(CAN3_FDC_VCU_PwrReq_OTA_Sta) -> [CAN3_FDC_VCU_PwrReq_OTA_Sta]
  FDCVCURWDRDCActiveSta/1(CAN3_FDC_VCU_RWDRDCActive_Sta) -> [CAN3_FDC_VCU_RWDRDCActive_Sta]
  FDCVCURegenTqLimitEnSta/1(CAN3_FDC_VCU_RegenTqLimitEn_Sta) -> [CAN3_FDC_VCU_RegenTqLimitEn_Sta]
  FDCVCUSlideRegenLimTqSta/1(CAN3_FDC_VCU_SlideRegenLimTq_Sta) -> [CAN3_FDC_VCU_SlideRegenLimTq_Sta]
  FDCVCUVehActSpdSta/1(CAN3_FDC_VCU_VehActSpd_Sta) -> [CAN3_FDC_VCU_VehActSpd_Sta]
  FDCVCUVehMalfunLevelSta/1(CAN3_FDC_VCU_VehMalfunLevel_Sta) -> [CAN3_FDC_VCU_VehMalfunLevel_Sta]
  FDCVMCActStESCYawSta/1(CAN3_FDC_VMC_ActStESCYaw_Sta) -> [CAN3_FDC_VMC_ActStESCYaw_Sta]
  FDCVMCLongAccSta/1(CAN3_FDC_VMC_LongAcc_Sta) -> [CAN3_FDC_VMC_LongAcc_Sta]
  FUSIONCMM1/1(CAN3_FUSION_CMM1) -> [CAN3_FUSION_CMM1]
  FUSIONCMM10/1(CAN3_FUSION_CMM10) -> [CAN3_FUSION_CMM10]
  FUSIONCMM2/1(CAN3_FUSION_CMM2) -> [CAN3_FUSION_CMM2]
  FUSIONCMM3/1(CAN3_FUSION_CMM3) -> [CAN3_FUSION_CMM3]
  FUSIONCMM4/1(CAN3_FUSION_CMM4) -> [CAN3_FUSION_CMM4]
  FUSIONCMM5/1(CAN3_FUSION_CMM5) -> [CAN3_FUSION_CMM5]
  FUSIONCMM6/1(CAN3_FUSION_CMM6) -> [CAN3_FUSION_CMM6]
  FUSIONCMM7/1(CAN3_FUSION_CMM7) -> [CAN3_FUSION_CMM7]
  FUSIONCMM8/1(CAN3_FUSION_CMM8) -> [CAN3_FUSION_CMM8]
  FUSIONCMM9/1(CAN3_FUSION_CMM9) -> [CAN3_FUSION_CMM9]
  FrTqSource/1(CAN3_Fr_TqSource) -> [CAN3_Fr_TqSource]
  HVRlyOpFail/1(CAN3_HVRlyOpFail) -> [CAN3_HVRlyOpFail]
  HVTHCMSysAvail/1(CAN3_HVTHCMSysAvail) -> [CAN3_HVTHCMSysAvail]
  LVBattChrgtimeAct/1(CAN3_LVBattChrgtimeAct) -> [CAN3_LVBattChrgtimeAct]
  LVBattVoltSta/1(CAN3_LVBattVoltSta) -> [CAN3_LVBattVoltSta]
  LVChrgHoldTAct/1(CAN3_LVChrgHoldTAct) -> [CAN3_LVChrgHoldTAct]
  LVSilentChrgLv/1(CAN3_LVSilentChrgLv) -> [CAN3_LVSilentChrgLv]
  LVSilentChrgReq/1(CAN3_LVSilentChrgReq) -> [CAN3_LVSilentChrgReq]
  LVSilentChrgSta/1(CAN3_LVSilentChrgSta) -> [CAN3_LVSilentChrgSta]
  MCUActDisFail/1(CAN3_MCUActDisFail) -> [CAN3_MCUActDisFail]
  PMMAllowECUSleep/1(CAN3_PMMAllowECUSleep) -> [CAN3_PMMAllowECUSleep]
  PmicBootReason/1(CAN3_PmicBootReason) -> [CAN3_PmicBootReason]
  PowerDownFault/1(CAN3_PowerDownFault) -> [CAN3_PowerDownFault]
  PowerDownState/1(CAN3_PowerDownState) -> [CAN3_PowerDownState]
  PowerUpFault/1(CAN3_PowerUpFault) -> [CAN3_PowerUpFault]
  PowerUpState/1(CAN3_PowerUpState) -> [CAN3_PowerUpState]
  PwrDownReq/1(CAN3_PwrDownReq) -> [CAN3_PwrDownReq]
  PwrStaConstraint/1(CAN3_PwrStaConstraint) -> [CAN3_PwrStaConstraint]
  PwrStaONTOIVIPopReq/1(CAN3_PwrStaONTOIVIPopReq) -> [CAN3_PwrStaONTOIVIPopReq]
  PwrStaONTOIVIPopT/1(CAN3_PwrStaONTOIVIPopT) -> [CAN3_PwrStaONTOIVIPopT]
  PwrStaSelect/1(CAN3_PwrStaSelect) -> [CAN3_PwrStaSelect]
  PwrStaTOSta/1(CAN3_PwrStaTOSta) -> [CAN3_PwrStaTOSta]
  PwrUpReq/1(CAN3_PwrUpReq) -> [CAN3_PwrUpReq]
  RrTqSource/1(CAN3_Rr_TqSource) -> [CAN3_Rr_TqSource]
  SchedChgTOSta/1(CAN3_SchedChgTOSta) -> [CAN3_SchedChgTOSta]
  SilentChkAllowSleep/1(CAN3_SilentChkAllowSleep) -> [CAN3_SilentChkAllowSleep]
  SysAllowReadySta/1(CAN3_SysAllowReadySta) -> [CAN3_SysAllowReadySta]
  SysPwrSta/1(CAN3_SysPwrSta) -> [CAN3_SysPwrSta]
  TCountSta/1(CAN3_TCountSta) -> [CAN3_TCountSta]
  TimerAllowSleep/1(CAN3_TimerAllowSleep) -> [CAN3_TimerAllowSleep]
  VCUBrkSWSta/1(CAN3_VCUBrkSWSta) -> [CAN3_VCUBrkSWSta]
  VCUFLDoorSta/1(CAN3_VCUFLDoorSta) -> [CAN3_VCUFLDoorSta]
  VCUFRDoorSta/1(CAN3_VCUFRDoorSta) -> [CAN3_VCUFRDoorSta]
  VCURLDoorSta/1(CAN3_VCURLDoorSta) -> [CAN3_VCURLDoorSta]
  VCURRDoorSta/1(CAN3_VCURRDoorSta) -> [CAN3_VCURRDoorSta]
  VehHVPwrAvail4THCM/1(CAN3_VehHVPwrAvail4THCM) -> [CAN3_VehHVPwrAvail4THCM]
  WisrBootReason/1(CAN3_WisrBootReason) -> [CAN3_WisrBootReason]
  bus_selector/1 -> EVCCAplusPwrUpReq/1(EVCCAplusPwrUpReq)  "<VOUTP_EvccAplusPwrUpReq_flg>"
  [BOUTP_outputs] -> bus_selector/1
  Ground/1 -> FDADC12VDet/1(FDADC12VDet)
  bus_selector1/1 -> FDADC12VDetAvg/1(FDADC12VDetAvg)  "<VOUTP_FDADC12VDetAvg_mV>"
  [BOUTP_outputs] -> bus_selector1/1
  Ground1/1 -> FDCVCUActMaxSlideRateSta/1(FDCVCUActMaxSlideRateSta)
  Ground2/1 -> FDCVCUAllowMovThdOTASta/1(FDCVCUAllowMovThdOTASta)
  Ground3/1 -> FDCVCUDTCCarouselSta/1(FDCVCUDTCCarouselSta)
  Ground4/1 -> FDCVCUForcePCmd/1(FDCVCUForcePCmd)
  Ground5/1 -> FDCVCUOTAPwrReqOFFChkSta/1(FDCVCUOTAPwrReqOFFChkSta)
  Ground6/1 -> FDCVCUOTAPwrReqStdChkSta/1(FDCVCUOTAPwrReqStdChkSta)
  Ground7/1 -> FDCVCUPwrReqOTASta/1(FDCVCUPwrReqOTASta)
  Ground8/1 -> FDCVCURWDRDCActiveSta/1(FDCVCURWDRDCActiveSta)
  Ground9/1 -> FDCVCURegenTqLimitEnSta/1(FDCVCURegenTqLimitEnSta)
  Ground10/1 -> FDCVCUSlideRegenLimTqSta/1(FDCVCUSlideRegenLimTqSta)
  Ground11/1 -> FDCVCUVehActSpdSta/1(FDCVCUVehActSpdSta)
  Ground12/1 -> FDCVCUVehMalfunLevelSta/1(FDCVCUVehMalfunLevelSta)
  Ground13/1 -> FDCVMCActStESCYawSta/1(FDCVMCActStESCYawSta)
  Ground14/1 -> FDCVMCLongAccSta/1(FDCVMCLongAccSta)
  Ground15/1 -> FUSIONCMM1/1(FUSIONCMM1)
  Ground16/1 -> FUSIONCMM10/1(FUSIONCMM10)
  Ground17/1 -> FUSIONCMM2/1(FUSIONCMM2)
  Ground18/1 -> FUSIONCMM3/1(FUSIONCMM3)
  Ground19/1 -> FUSIONCMM4/1(FUSIONCMM4)
  Ground20/1 -> FUSIONCMM5/1(FUSIONCMM5)
  Ground21/1 -> FUSIONCMM6/1(FUSIONCMM6)
  Ground22/1 -> FUSIONCMM7/1(FUSIONCMM7)
  Ground23/1 -> FUSIONCMM8/1(FUSIONCMM8)
  Ground24/1 -> FUSIONCMM9/1(FUSIONCMM9)
  Ground25/1 -> FrTqSource/1(FrTqSource)
  Ground26/1 -> HVRlyOpFail/1(HVRlyOpFail)
  bus_selector2/1 -> HVTHCMSysAvail/1(HVTHCMSysAvail)  "<VOUTP_HVTHCMSysAvail_enum>"
  [BOUTP_outputs] -> bus_selector2/1
  bus_selector3/1 -> LVBattChrgtimeAct/1(LVBattChrgtimeAct)  "<VOUTP_LVBattChrgTimeCnt_s>"
  [BOUTP_outputs] -> bus_selector3/1
  bus_selector4/1 -> LVBattVoltSta/1(LVBattVoltSta)  "<VOUTP_LVBattVoltSta_enum>"
  [BOUTP_outputs] -> bus_selector4/1
  bus_selector5/1 -> LVChrgHoldTAct/1(LVChrgHoldTAct)  "<VOUTP_LVChrgHoldTtimer_s>"
  [BOUTP_outputs] -> bus_selector5/1
  bus_selector6/1 -> LVSilentChrgLv/1(LVSilentChrgLv)  "<VOUTP_LVSilentChrgLv_enum>"
  [BOUTP_outputs] -> bus_selector6/1
  bus_selector7/1 -> LVSilentChrgReq/1(LVSilentChrgReq)  "<VOUTP_LVSilentChrgReq_flg>"
  [BOUTP_outputs] -> bus_selector7/1
  bus_selector8/1 -> LVSilentChrgSta/1(LVSilentChrgSta)  "<VOUTP_LVSilentChrgSta_enum>"
  [BOUTP_outputs] -> bus_selector8/1
  Ground27/1 -> MCUActDisFail/1(MCUActDisFail)
  bus_selector9/1 -> PMMAllowECUSleep/1(PMMAllowECUSleep)  "<VOUTP_PMMAllowECUSleep_flg>"
  [BOUTP_outputs] -> bus_selector9/1
  bus_selector10/1 -> PmicBootReason/1(PmicBootReason)  "<VOUTP_PmicBootReason_enum>"
  [BOUTP_outputs] -> bus_selector10/1
  bus_selector11/1 -> PowerDownFault/1(PowerDownFault)  "<VOUTP_PowerDownFault_enum>"
  [BOUTP_outputs] -> bus_selector11/1
  bus_selector12/1 -> PowerDownState/1(PowerDownState)  "<VOUTP_PowerDownState_enum>"
  [BOUTP_outputs] -> bus_selector12/1
  bus_selector13/1 -> PowerUpFault/1(PowerUpFault)  "<VOUTP_PowerUpFault_enum>"
  [BOUTP_outputs] -> bus_selector13/1
  bus_selector14/1 -> PowerUpState/1(PowerUpState)  "<VOUTP_PowerUpState_enum>"
  [BOUTP_outputs] -> bus_selector14/1
  bus_selector15/1 -> PwrDownReq/1(PwrDownReq)  "<VOUTP_PwrDownReq_enum>"
  [BOUTP_outputs] -> bus_selector15/1
  bus_selector16/1 -> PwrStaConstraint/1(PwrStaConstraint)  "<VOUTP_PwrStaConstraint_enum>"
  [BOUTP_outputs] -> bus_selector16/1
  bus_selector17/1 -> PwrStaONTOIVIPopReq/1(PwrStaONTOIVIPopReq)  "<VOUTP_PwrStaONTOPopReq_flg>"
  [BOUTP_outputs] -> bus_selector17/1
  bus_selector18/1 -> PwrStaONTOIVIPopT/1(PwrStaONTOIVIPopT)  "<VOUTP_IVIPwrStaONTOPopT_s>"
  [BOUTP_outputs] -> bus_selector18/1
  bus_selector19/1 -> PwrStaSelect/1(PwrStaSelect)  "<VOUTP_PwrStaSelect_enum>"
  [BOUTP_outputs] -> bus_selector19/1
  bus_selector20/1 -> PwrStaTOSta/1(PwrStaTOSta)  "<VOUTP_PwrStaTOSta_enum>"
  [BOUTP_outputs] -> bus_selector20/1
  bus_selector21/1 -> PwrUpReq/1(PwrUpReq)  "<VOUTP_PwrUpReq_enum>"
  [BOUTP_outputs] -> bus_selector21/1
  bus_selector22/1 -> RrTqSource/1(RrTqSource)  "<VOUTP_TqSourceRr_enum>"
  [BOUTP_outputs] -> bus_selector22/1
  Ground28/1 -> SchedChgTOSta/1(SchedChgTOSta)
  bus_selector23/1 -> SilentChkAllowSleep/1(SilentChkAllowSleep)  "<VOUTP_SilentChkAllowSleep_flg>"
  [BOUTP_outputs] -> bus_selector23/1
  Ground29/1 -> SysAllowReadySta/1(SysAllowReadySta)
  bus_selector24/1 -> SysPwrSta/1(SysPwrSta)  "<VOUTP_SysPowerMode_enum>"
  [BOUTP_outputs] -> bus_selector24/1
  bus_selector25/1 -> TCountSta/1(TCountSta)  "<VOUTP_TCountSta_enum>"
  [BOUTP_outputs] -> bus_selector25/1
  bus_selector26/1 -> TimerAllowSleep/1(TimerAllowSleep)  "<VOUTP_TimerAllowSleep_flg>"
  [BOUTP_outputs] -> bus_selector26/1
  Ground30/1 -> VCUBrkSWSta/1(VCUBrkSWSta)
  Ground31/1 -> VCUFLDoorSta/1(VCUFLDoorSta)
  Ground32/1 -> VCUFRDoorSta/1(VCUFRDoorSta)
  Ground33/1 -> VCURLDoorSta/1(VCURLDoorSta)
  Ground34/1 -> VCURRDoorSta/1(VCURRDoorSta)
  Ground35/1 -> WisrBootReason/1(WisrBootReason)
  Ground36/1 -> Data Type Conversion1/1
  s8_AcoreReadyToSleep/1 -> Subsystem/1(s8_AcoreReadyToSleep)
  Data Type Conversion1/1 -> Subsystem/3(VOUTP_OTAPwrReqOFFChkSta_enum)
  [BOUTP_outputs] -> bus_selector28/1
  Data Type Conversion2/1 -> Subsystem/4(VOUTP_OTAPwrReqStdChkSta_enum)
  Ground37/1 -> Data Type Conversion2/1
  Data Type Conversion/1 -> Subsystem/2(VOUTP_CurrentNmState_enum)
  bus_selector28/1 -> Data Type Conversion/1  "<VOUTP_CurrentNmState_enum>"
  Subsystem/1(VehHVPwrAvail4THCM) -> VehHVPwrAvail4THCM/1(VehHVPwrAvail4THCM)

== system halout/HAL_OUT/CAN3/FD3_VCU1_0x115 ==
  BSCP_outputs : Inport  OutDataTypeStr=Bus: BSCP_outputs
  BOUTP_outputs : Inport  Port=2  OutDataTypeStr=Bus: BOUTP_outputs
  ActiveDischReq : Subsystem
  CSVCU1 : Subsystem
  CoastDwModeStaChk : Subsystem
  DCDCEnaReq : Subsystem
  DCDCVoltSetpoint : Subsystem
  DemoModeStaChk : Subsystem
  DrSeatSta : Subsystem
  DynoModeStaChk : Subsystem
  Ground{,1..8} (9 alike) : Ground
  HVBatCnctReq : Subsystem
  HVSysReadyToCharge : Subsystem
  LVChrgFuncStaChk : Subsystem
  MSACrlSta : Subsystem
  PButtonSta : Subsystem
  PrkReq : Subsystem
  PrkReqValid : Subsystem
  PwrSta : Subsystem
  RCVCU1 : Subsystem
  ShiftGearPosn : Subsystem
  bus_creator : BusCreator  Inputs=18  OutDataTypeStr=Bus: DT_CAN3_SG_FD3_VCU1  NonVirtualBus=on
  bus_selector : BusSelector  OutputSignals=VOUTP_ActiveDischargeReq_flg
  bus_selector1 : BusSelector  OutputSignals=VOUTP_DCDCEnaReq_flg
  bus_selector2 : BusSelector  OutputSignals=VOUTP_DCDCVoltSetpoint_V
  bus_selector3 : BusSelector  OutputSignals=VOUTP_DrSeatSta_enum
  bus_selector4 : BusSelector  OutputSignals=VOUTP_HVBatCnctReq_flg
  bus_selector5 : BusSelector  OutputSignals=VOUTP_HVSysReadyToCharge_enum
  bus_selector6 : BusSelector  OutputSignals=VOUTP_MSACtrlSta_enum
  bus_selector7 : BusSelector  OutputSignals=VOUTP_PowerSta_enum
  bus_selector8 : BusSelector  OutputSignals=VOUTP_ShiftGearPosn_enum
  FD3_VCU1 : Outport
  wires:
  BSCP_outputs/1 -> [BSCP_outputs]
  BOUTP_outputs/1 -> [BOUTP_outputs]
  [CAN3_ActiveDischReq] -> bus_creator/1  "CAN3_ActiveDischReq"
  [CAN3_CS_VCU1] -> bus_creator/2  "CAN3_CS_VCU1"
  [CAN3_CoastDwModeStaChk] -> bus_creator/3  "CAN3_CoastDwModeStaChk"
  [CAN3_DCDCEnaReq] -> bus_creator/4  "CAN3_DCDCEnaReq"
  [CAN3_DCDCVoltSetpoint] -> bus_creator/5  "CAN3_DCDCVoltSetpoint"
  [CAN3_DemoModeStaChk] -> bus_creator/6  "CAN3_DemoModeStaChk"
  [CAN3_Dr_SeatSta] -> bus_creator/7  "CAN3_Dr_SeatSta"
  [CAN3_DynoModeStaChk] -> bus_creator/8  "CAN3_DynoModeStaChk"
  [CAN3_HVBatCnctReq] -> bus_creator/9  "CAN3_HVBatCnctReq"
  [CAN3_HVSysReadyToCharge] -> bus_creator/10  "CAN3_HVSysReadyToCharge"
  [CAN3_LVChrgFuncStaChk] -> bus_creator/11  "CAN3_LVChrgFuncStaChk"
  [CAN3_MSA_Crl_Sta] -> bus_creator/12  "CAN3_MSA_Crl_Sta"
  [CAN3_P_Button_Sta] -> bus_creator/13  "CAN3_P_Button_Sta"
  [CAN3_PrkReq] -> bus_creator/14  "CAN3_PrkReq"
  [CAN3_PrkReqValid] -> bus_creator/15  "CAN3_PrkReqValid"
  [CAN3_PwrSta] -> bus_creator/16  "CAN3_PwrSta"
  [CAN3_RC_VCU1] -> bus_creator/17  "CAN3_RC_VCU1"
  [CAN3_ShiftGearPosn] -> bus_creator/18  "CAN3_ShiftGearPosn"
  bus_creator/1 -> FD3_VCU1/1
  ActiveDischReq/1(CAN3_ActiveDischReq) -> [CAN3_ActiveDischReq]
  CSVCU1/1(CAN3_CS_VCU1) -> [CAN3_CS_VCU1]
  CoastDwModeStaChk/1(CAN3_CoastDwModeStaChk) -> [CAN3_CoastDwModeStaChk]
  DCDCEnaReq/1(CAN3_DCDCEnaReq) -> [CAN3_DCDCEnaReq]
  DCDCVoltSetpoint/1(CAN3_DCDCVoltSetpoint) -> [CAN3_DCDCVoltSetpoint]
  DemoModeStaChk/1(CAN3_DemoModeStaChk) -> [CAN3_DemoModeStaChk]
  DrSeatSta/1(CAN3_Dr_SeatSta) -> [CAN3_Dr_SeatSta]
  DynoModeStaChk/1(CAN3_DynoModeStaChk) -> [CAN3_DynoModeStaChk]
  HVBatCnctReq/1(CAN3_HVBatCnctReq) -> [CAN3_HVBatCnctReq]
  HVSysReadyToCharge/1(CAN3_HVSysReadyToCharge) -> [CAN3_HVSysReadyToCharge]
  LVChrgFuncStaChk/1(CAN3_LVChrgFuncStaChk) -> [CAN3_LVChrgFuncStaChk]
  MSACrlSta/1(CAN3_MSA_Crl_Sta) -> [CAN3_MSA_Crl_Sta]
  PButtonSta/1(CAN3_P_Button_Sta) -> [CAN3_P_Button_Sta]
  PrkReq/1(CAN3_PrkReq) -> [CAN3_PrkReq]
  PrkReqValid/1(CAN3_PrkReqValid) -> [CAN3_PrkReqValid]
  PwrSta/1(CAN3_PwrSta) -> [CAN3_PwrSta]
  RCVCU1/1(CAN3_RC_VCU1) -> [CAN3_RC_VCU1]
  ShiftGearPosn/1(CAN3_ShiftGearPosn) -> [CAN3_ShiftGearPosn]
  bus_selector/1 -> ActiveDischReq/1(ActiveDischReq)  "<VOUTP_ActiveDischargeReq_flg>"
  [BOUTP_outputs] -> bus_selector/1
  Ground/1 -> CSVCU1/1(CSVCU1)
  Ground1/1 -> CoastDwModeStaChk/1(CoastDwModeStaChk)
  bus_selector1/1 -> DCDCEnaReq/1(DCDCEnaReq)  "<VOUTP_DCDCEnaReq_flg>"
  [BOUTP_outputs] -> bus_selector1/1
  bus_selector2/1 -> DCDCVoltSetpoint/1(DCDCVoltSetpoint)  "<VOUTP_DCDCVoltSetpoint_V>"
  [BOUTP_outputs] -> bus_selector2/1
  Ground2/1 -> DemoModeStaChk/1(DemoModeStaChk)
  bus_selector3/1 -> DrSeatSta/1(DrSeatSta)  "<VOUTP_DrSeatSta_enum>"
  [BOUTP_outputs] -> bus_selector3/1
  Ground3/1 -> DynoModeStaChk/1(DynoModeStaChk)
  bus_selector4/1 -> HVBatCnctReq/1(HVBatCnctReq)  "<VOUTP_HVBatCnctReq_flg>"
  [BOUTP_outputs] -> bus_selector4/1
  bus_selector5/1 -> HVSysReadyToCharge/1(HVSysReadyToCharge)  "<VOUTP_HVSysReadyToCharge_enum>"
  [BOUTP_outputs] -> bus_selector5/1
  Ground4/1 -> LVChrgFuncStaChk/1(LVChrgFuncStaChk)
  bus_selector6/1 -> MSACrlSta/1(MSACrlSta)  "<VOUTP_MSACtrlSta_enum>"
  [BOUTP_outputs] -> bus_selector6/1
  Ground5/1 -> PButtonSta/1(PButtonSta)
  Ground6/1 -> PrkReq/1(PrkReq)
  Ground7/1 -> PrkReqValid/1(PrkReqValid)
  bus_selector7/1 -> PwrSta/1(PwrSta)  "<VOUTP_PowerSta_enum>"
  [BOUTP_outputs] -> bus_selector7/1
  Ground8/1 -> RCVCU1/1(RCVCU1)
  bus_selector8/1 -> ShiftGearPosn/1(ShiftGearPosn)  "<VOUTP_ShiftGearPosn_enum>"
  [BOUTP_outputs] -> bus_selector8/1

== system halout/HAL_OUT/CAN3/FD3_VCU1_Tx ==
  TxReq : Inport
  BSCP_outputs : Inport  Port=2  OutDataTypeStr=Bus: BSCP_outputs
  BOUTP_outputs : Inport  Port=3  OutDataTypeStr=Bus: BOUTP_outputs
  Chart : Stateflow chart  TreatAsAtomicUnit=on
  Constant : Constant  Value=C_TASK_5MS_S
  Constant3 : Constant  Value=CycleTime
  Data Type Conversion : DataTypeConversion  OutDataTypeStr=uint16
  Data Type Conversion1 : DataTypeConversion  OutDataTypeStr=uint8
  Divide : Product  Inputs=*/
  Gain : Gain  Gain=0.001
  Ground{,1..8} (9 alike) : Ground
  OR : Logic  Operator=OR  Inputs=18  AllPortsSameDT=off  OutDataTypeStr=boolean
  bus_selector : BusSelector  OutputSignals=VOUTP_ActiveDischargeReq_flg
  bus_selector1 : BusSelector  OutputSignals=VOUTP_DCDCEnaReq_flg
  bus_selector2 : BusSelector  OutputSignals=VOUTP_DCDCVoltSetpoint_V
  bus_selector3 : BusSelector  OutputSignals=VOUTP_DrSeatSta_enum
  bus_selector4 : BusSelector  OutputSignals=VOUTP_HVBatCnctReq_flg
  bus_selector5 : BusSelector  OutputSignals=VOUTP_HVSysReadyToCharge_enum
  bus_selector6 : BusSelector  OutputSignals=VOUTP_MSACtrlSta_enum
  bus_selector7 : BusSelector  OutputSignals=VOUTP_PowerSta_enum
  bus_selector8 : BusSelector  OutputSignals=VOUTP_ShiftGearPosn_enum
  convert_out : FVT_lib/hal/convert_out  gain=0.0235  offset=12
  detect_change{,1..8} (9 alike) : simulink/Logic and Bit Operations/Detect Change  vinit=0  OutDataTypeStr=boolean
  TxTrigger : Outport
  wires:
  Data Type Conversion/1 -> Chart/3(CycleCnt)
  TxReq/1 -> Chart/1(TxReq)
  [EventReq_flg] -> Chart/2(EventReq)
  Constant/1 -> Divide/2
  Divide/1 -> Data Type Conversion/1
  Chart/1(TxTrigger) -> TxTrigger/1
  Gain/1 -> Divide/1
  Constant3/1 -> Gain/1
  BSCP_outputs/1 -> [BSCP_outputs]
  BOUTP_outputs/1 -> [BOUTP_outputs]
  OR/1 -> [EventReq_flg]
  detect_change/1 -> OR/1
  bus_selector/1 -> detect_change/1  "<VOUTP_ActiveDischargeReq_flg>"
  [BOUTP_outputs] -> bus_selector/1
  Ground/1 -> OR/2
  Ground1/1 -> OR/3
  detect_change1/1 -> OR/4
  bus_selector1/1 -> detect_change1/1  "<VOUTP_DCDCEnaReq_flg>"
  [BOUTP_outputs] -> bus_selector1/1
  detect_change2/1 -> OR/5
  Data Type Conversion1/1 -> detect_change2/1
  convert_out/1 -> Data Type Conversion1/1
  bus_selector2/1 -> convert_out/1  "<VOUTP_DCDCVoltSetpoint_V>"
  [BOUTP_outputs] -> bus_selector2/1
  Ground2/1 -> OR/6
  detect_change3/1 -> OR/7
  bus_selector3/1 -> detect_change3/1  "<VOUTP_DrSeatSta_enum>"
  [BOUTP_outputs] -> bus_selector3/1
  Ground3/1 -> OR/8
  detect_change4/1 -> OR/9
  bus_selector4/1 -> detect_change4/1  "<VOUTP_HVBatCnctReq_flg>"
  [BOUTP_outputs] -> bus_selector4/1
  detect_change5/1 -> OR/10
  bus_selector5/1 -> detect_change5/1  "<VOUTP_HVSysReadyToCharge_enum>"
  [BOUTP_outputs] -> bus_selector5/1
  Ground4/1 -> OR/11
  detect_change6/1 -> OR/12
  bus_selector6/1 -> detect_change6/1  "<VOUTP_MSACtrlSta_enum>"
  [BOUTP_outputs] -> bus_selector6/1
  Ground5/1 -> OR/13
  Ground6/1 -> OR/14
  Ground7/1 -> OR/15
  detect_change7/1 -> OR/16
  bus_selector7/1 -> detect_change7/1  "<VOUTP_PowerSta_enum>"
  [BOUTP_outputs] -> bus_selector7/1
  Ground8/1 -> OR/17
  detect_change8/1 -> OR/18
  bus_selector8/1 -> detect_change8/1  "<VOUTP_ShiftGearPosn_enum>"
  [BOUTP_outputs] -> bus_selector8/1
